simulink model "Clik_Jacobian_inverse_corrado"  (R2023b)
settings: Solver=VariableStepAuto  StartTime=0.0  StopTime=20  RelTol=1e-3
model workspace: external: MAT-File (data not in the file)
undefined symbols (not defined in the file): DiscIntNeverNeededParam, f_s
settings Model: Creator=benit  LastModifiedBy=lalla
settings OptimizationCC: ReuseModelBlockBuffer=off

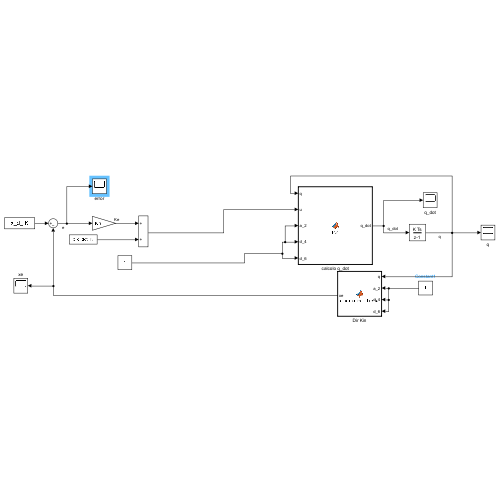
[thumbnail: Simulink's stored preview of the top-level diagram]
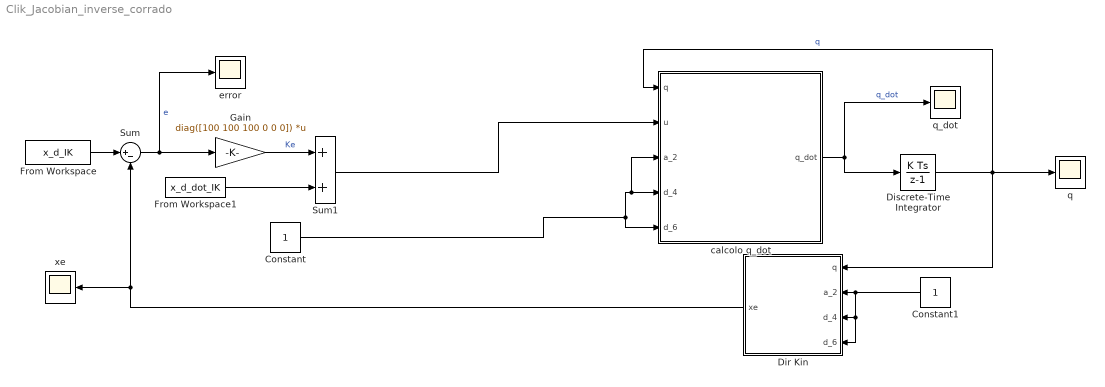
== system Clik_Jacobian_inverse_corrado ==
  Constant : Constant
  Constant1 : Constant
  Dir Kin : MATLAB Function  TreatAsAtomicUnit=on
  Discrete-Time Integrator : DiscreteIntegrator  gainval=1  InitialCondition=[0,0,0,0,0,0]'  SampleTime=1/f_s  ICPrevOutput=DiscIntNeverNeededParam  ICPrevScaledInput=DiscIntNeverNeededParam
  From Workspace : FromWorkspace  VariableName=x_d_IK
  From Workspace1 : FromWorkspace  VariableName=x_d_dot_IK
  Gain : Gain  Gain=diag([100 100 100 0 0 0])  Multiplication=Matrix(K*u)
  Sum : Sum  Inputs=|+-
  Sum1 : Sum
  calcolo q_dot : MATLAB Function  TreatAsAtomicUnit=on
  error : Scope
  q : Scope
  q_dot : Scope
  xe : Scope
  wires:
  Gain/1 -> Sum1/1  "Ke"
  Sum/1 -> error/1, Gain/1  "e"
  From Workspace/1 -> Sum/1
  Discrete-Time Integrator/1 -> q/1, Dir Kin/1(q), calcolo q_dot/1(q)  "q"
  calcolo q_dot/1(q_dot) -> q_dot/1, Discrete-Time Integrator/1  "q_dot"
  Sum1/1 -> calcolo q_dot/2(u)
  Dir Kin/1(xe) -> xe/1, Sum/2
  From Workspace1/1 -> Sum1/2
  Constant/1 -> calcolo q_dot/3(a_2), calcolo q_dot/4(d_4), calcolo q_dot/5(d_6)
  Constant1/1 -> Dir Kin/4(d_6), Dir Kin/3(d_4), Dir Kin/2(a_2)

== matlab function Clik_Jacobian_inverse_corrado/calcolo q_dot ==
  data: q input; u input; a_2 input; d_4 input; q_dot output; d_6 input
function q_dot = fcn(q,u,a_2,d_4,d_6)


theta_1 =q(1);
theta_2 =q(2);
theta_3 =q(3);
theta_4 =q(4);
theta_5 =q(5);
theta_6 =q(6);

    J = [  - d_4*(cos(theta_2)*sin(theta_1)*sin(theta_3) - cos(theta_3)*sin(theta_1)*sin(theta_2)) - d_6*(sin(theta_5)*(cos(theta_1)*sin(theta_4) - cos(theta_4)*(sin(theta_1)*sin(theta_2)*sin(theta_3) - cos(theta_2)*cos(theta_3)*sin(theta_1))) - cos(theta_5)*(cos(theta_2)*sin(theta_1)*sin(theta_3) - cos(theta_3)*sin(theta_1)*sin(theta_2))) - a_2*cos(theta_2)*sin(theta_1),                                                                                           cos(theta_1)*(a_2*sin(theta_2) + d_4*cos(theta_2 - theta_3) + (d_6*sin(theta_2 + theta_3)*sin(theta_4 + theta_5))/2 - (d_6*sin(theta_4 - theta_5)*sin(theta_2 + theta_3))/2 - d_6*cos(theta_2 - theta_3)*cos(theta_5)),                                                                                           cos(theta_1)*(d_4*cos(theta_2 - theta_3) + (d_6*sin(theta_2 + theta_3)*sin(theta_4 + theta_5))/2 - (d_6*sin(theta_4 - theta_5)*sin(theta_2 + theta_3))/2 - d_6*cos(theta_2 - theta_3)*cos(theta_5)), -d_6*sin(theta_5)*(2*cos(theta_3)^2*cos(theta_4)*sin(theta_1) - cos(theta_4)*sin(theta_1) + cos(theta_1)*cos(theta_2)*cos(theta_3)*sin(theta_4) + cos(theta_1)*sin(theta_2)*sin(theta_3)*sin(theta_4)), d_6*cos(theta_1)*cos(theta_2)*sin(theta_3)*sin(theta_5) - d_6*cos(theta_5)*sin(theta_1)*sin(theta_4) + d_6*cos(theta_1)*cos(theta_3)*sin(theta_2)*sin(theta_5) + 2*d_6*cos(theta_3)^2*cos(theta_5)*sin(theta_1)*sin(theta_4) + d_6*cos(theta_1)*cos(theta_4)*cos(theta_5)*sin(theta_2)*sin(theta_3) - 2*d_6*cos(theta_1)*cos(theta_2)*cos(theta_4)^2*sin(theta_3)*sin(theta_5) - 2*d_6*cos(theta_1)*cos(theta_3)*cos(theta_4)^2*sin(theta_2)*sin(theta_5) + d_6*cos(theta_1)*cos(theta_2)*cos(theta_3)*cos(theta_4)*cos(theta_5),                                                                                                                                                                                                                           0;
            d_6*(sin(theta_5)*(sin(theta_1)*sin(theta_4) - cos(theta_4)*(cos(theta_1)*sin(theta_2)*sin(theta_3) - cos(theta_1)*cos(theta_2)*cos(theta_3))) - cos(theta_5)*(cos(theta_1)*cos(theta_2)*sin(theta_3) - cos(theta_1)*cos(theta_3)*sin(theta_2))) + d_4*(cos(theta_1)*cos(theta_2)*sin(theta_3) - cos(theta_1)*cos(theta_3)*sin(theta_2)) + a_2*cos(theta_1)*cos(theta_2),                                                                                          -sin(theta_1)*(a_2*sin(theta_2) + d_4*cos(theta_2 - theta_3) + (d_6*sin(theta_2 + theta_3)*sin(theta_4 + theta_5))/2 - (d_6*sin(theta_4 - theta_5)*sin(theta_2 + theta_3))/2 - d_6*cos(theta_2 - theta_3)*cos(theta_5)),                                                                                          -sin(theta_1)*(d_4*cos(theta_2 - theta_3) + (d_6*sin(theta_2 + theta_3)*sin(theta_4 + theta_5))/2 - (d_6*sin(theta_4 - theta_5)*sin(theta_2 + theta_3))/2 - d_6*cos(theta_2 - theta_3)*cos(theta_5)),  d_6*sin(theta_5)*(2*cos(theta_1)*cos(theta_3)^2*cos(theta_4) - cos(theta_1)*cos(theta_4) + cos(theta_2)*cos(theta_3)*sin(theta_1)*sin(theta_4) + sin(theta_1)*sin(theta_2)*sin(theta_3)*sin(theta_4)), d_6*cos(theta_1)*cos(theta_5)*sin(theta_4) - d_6*cos(theta_2)*sin(theta_1)*sin(theta_3)*sin(theta_5) - d_6*cos(theta_3)*sin(theta_1)*sin(theta_2)*sin(theta_5) - 2*d_6*cos(theta_1)*cos(theta_3)^2*cos(theta_5)*sin(theta_4) - d_6*cos(theta_2)*cos(theta_3)*cos(theta_4)*cos(theta_5)*sin(theta_1) - d_6*cos(theta_4)*cos(theta_5)*sin(theta_1)*sin(theta_2)*sin(theta_3) + 2*d_6*cos(theta_2)*cos(theta_4)^2*sin(theta_1)*sin(theta_3)*sin(theta_5) + 2*d_6*cos(theta_3)*cos(theta_4)^2*sin(theta_1)*sin(theta_2)*sin(theta_5),                                                                                                                                                                                                                             0;
                                                                                                                                                                                                                                                                                                                                                                        0, -cos(2*theta_1)*(a_2*cos(theta_2) + d_4*cos(theta_2)*sin(theta_3) - d_4*cos(theta_3)*sin(theta_2) - d_6*cos(theta_2)*cos(theta_5)*sin(theta_3) + d_6*cos(theta_3)*cos(theta_5)*sin(theta_2) + d_6*cos(theta_2)*cos(theta_3)*cos(theta_4)*sin(theta_5) - d_6*cos(theta_4)*sin(theta_2)*sin(theta_3)*sin(theta_5)), -cos(2*theta_1)*(d_4*cos(theta_2)*sin(theta_3) - d_4*cos(theta_3)*sin(theta_2) - d_6*cos(theta_2)*cos(theta_5)*sin(theta_3) + d_6*cos(theta_3)*cos(theta_5)*sin(theta_2) + d_6*cos(theta_2)*cos(theta_3)*cos(theta_4)*sin(theta_5) - d_6*cos(theta_4)*sin(theta_2)*sin(theta_3)*sin(theta_5)),                                                                                                                                   -d_6*sin(theta_2 - theta_3)*cos(2*theta_1)*sin(theta_4)*sin(theta_5),                                                                                                                                                                                             d_6*cos(2*theta_1)*(sin(theta_2)*sin(theta_3)*sin(theta_5) - cos(theta_2)*cos(theta_3)*sin(theta_5) + 2*cos(theta_2)*cos(theta_3)*cos(theta_4)^2*sin(theta_5) - 2*cos(theta_4)^2*sin(theta_2)*sin(theta_3)*sin(theta_5) - cos(theta_2)*cos(theta_4)*cos(theta_5)*sin(theta_3) + cos(theta_3)*cos(theta_4)*cos(theta_5)*sin(theta_2)),                                                                                                                                                                                                                                          0;
                                                                                                                                                                                                                                                                                                                                                              0,                                                                                                                                                                                                                                                                                                     sin(theta_1),                                                                                                                                                                                                                                                                                  sin(theta_1),                                                                                                                                                                   -sin(theta_2 - theta_3)*cos(theta_1),                                                                                                                                                                                                                                                                                                                                                                                                       sin(theta_4)*(cos(theta_1)*sin(theta_2)*sin(theta_3) - cos(theta_1)*cos(theta_2)*cos(theta_3)) - cos(theta_4)*sin(theta_1), sin(theta_5)*(sin(theta_1)*sin(theta_4) - cos(theta_4)*(cos(theta_1)*sin(theta_2)*sin(theta_3) - cos(theta_1)*cos(theta_2)*cos(theta_3))) - cos(theta_5)*(cos(theta_1)*cos(theta_2)*sin(theta_3) - cos(theta_1)*cos(theta_3)*sin(theta_2));
                                                                                                                                                                                                                                                                                                                                                                         0,                                                                                                                                                                                                                                                                                                     cos(theta_1),                                                                                                                                                                                                                                                                                  cos(theta_1),                                                                                                                                                                   -sin(theta_2 - theta_3)*sin(theta_1),                                                                                                                                                                                                                                                                                                                                                                                                       sin(theta_4)*(sin(theta_1)*sin(theta_2)*sin(theta_3) - cos(theta_2)*cos(theta_3)*sin(theta_1)) - cos(theta_1)*cos(theta_4), sin(theta_5)*(cos(theta_1)*sin(theta_4) - cos(theta_4)*(sin(theta_1)*sin(theta_2)*sin(theta_3) - cos(theta_2)*cos(theta_3)*sin(theta_1))) - cos(theta_5)*(cos(theta_2)*sin(theta_1)*sin(theta_3) - cos(theta_3)*sin(theta_1)*sin(theta_2));
                                                                                                                                                                                                                                                                                                                                                              1,                                                                                                                                                                                                                                                                                                                0,                                                                                                                                                                                                                                                                                             0,                                                                                                                                                                                 cos(theta_2 - theta_3),                                                                                                                                                                                                                                                                                                                                                                                                                                                                                             -sin(theta_2 + theta_3)*sin(theta_4),                                                                                                                                                     sin(theta_2 + theta_3)*cos(theta_4)*sin(theta_5) - cos(theta_2 - theta_3)*cos(theta_5)];
 
    q_dot = pinv(J)*u;

end

== matlab function Clik_Jacobian_inverse_corrado/Dir Kin ==
  data: q input; xe output; a_2 input; d_4 input; d_6 input
function xe = cinematica_diretta(q,a_2,d_4,d_6)
 
theta_1 =q(1);
theta_2 =q(2);
theta_3 =q(3);
theta_4 =q(4);
theta_5 =q(5);
theta_6 =q(6);


Te=[cos(theta_6)*(cos(theta_5)*(sin(theta_1)*sin(theta_4) - cos(theta_4)*(cos(theta_1)*sin(theta_2)*sin(theta_3) - cos(theta_1)*cos(theta_2)*cos(theta_3))) - sin(theta_5)*(cos(theta_1)*cos(theta_2)*sin(theta_3) - cos(theta_1)*cos(theta_3)*sin(theta_2))) - sin(theta_6)*(cos(theta_4)*sin(theta_1) - sin(theta_4)*(cos(theta_1)*sin(theta_2)*sin(theta_3) - cos(theta_1)*cos(theta_2)*cos(theta_3))), - cos(theta_6)*(cos(theta_4)*sin(theta_1) - sin(theta_4)*(cos(theta_1)*sin(theta_2)*sin(theta_3) - cos(theta_1)*cos(theta_2)*cos(theta_3))) - sin(theta_6)*(cos(theta_5)*(sin(theta_1)*sin(theta_4) - cos(theta_4)*(cos(theta_1)*sin(theta_2)*sin(theta_3) - cos(theta_1)*cos(theta_2)*cos(theta_3))) - sin(theta_5)*(cos(theta_1)*cos(theta_2)*sin(theta_3) - cos(theta_1)*cos(theta_3)*sin(theta_2))), sin(theta_5)*(sin(theta_1)*sin(theta_4) - cos(theta_4)*(cos(theta_1)*sin(theta_2)*sin(theta_3) - cos(theta_1)*cos(theta_2)*cos(theta_3))) - cos(theta_5)*(cos(theta_1)*cos(theta_2)*sin(theta_3) - cos(theta_1)*cos(theta_3)*sin(theta_2)), d_6*(sin(theta_5)*(sin(theta_1)*sin(theta_4) - cos(theta_4)*(cos(theta_1)*sin(theta_2)*sin(theta_3) - cos(theta_1)*cos(theta_2)*cos(theta_3))) - cos(theta_5)*(cos(theta_1)*cos(theta_2)*sin(theta_3) - cos(theta_1)*cos(theta_3)*sin(theta_2))) + d_4*(cos(theta_1)*cos(theta_2)*sin(theta_3) - cos(theta_1)*cos(theta_3)*sin(theta_2)) + a_2*cos(theta_1)*cos(theta_2);
    cos(theta_6)*(cos(theta_5)*(cos(theta_1)*sin(theta_4) - cos(theta_4)*(sin(theta_1)*sin(theta_2)*sin(theta_3) - cos(theta_2)*cos(theta_3)*sin(theta_1))) - sin(theta_5)*(cos(theta_2)*sin(theta_1)*sin(theta_3) - cos(theta_3)*sin(theta_1)*sin(theta_2))) - sin(theta_6)*(cos(theta_1)*cos(theta_4) - sin(theta_4)*(sin(theta_1)*sin(theta_2)*sin(theta_3) - cos(theta_2)*cos(theta_3)*sin(theta_1))), - cos(theta_6)*(cos(theta_1)*cos(theta_4) - sin(theta_4)*(sin(theta_1)*sin(theta_2)*sin(theta_3) - cos(theta_2)*cos(theta_3)*sin(theta_1))) - sin(theta_6)*(cos(theta_5)*(cos(theta_1)*sin(theta_4) - cos(theta_4)*(sin(theta_1)*sin(theta_2)*sin(theta_3) - cos(theta_2)*cos(theta_3)*sin(theta_1))) - sin(theta_5)*(cos(theta_2)*sin(theta_1)*sin(theta_3) - cos(theta_3)*sin(theta_1)*sin(theta_2))), sin(theta_5)*(cos(theta_1)*sin(theta_4) - cos(theta_4)*(sin(theta_1)*sin(theta_2)*sin(theta_3) - cos(theta_2)*cos(theta_3)*sin(theta_1))) - cos(theta_5)*(cos(theta_2)*sin(theta_1)*sin(theta_3) - cos(theta_3)*sin(theta_1)*sin(theta_2)), d_4*(cos(theta_2)*sin(theta_1)*sin(theta_3) - cos(theta_3)*sin(theta_1)*sin(theta_2)) + d_6*(sin(theta_5)*(cos(theta_1)*sin(theta_4) - cos(theta_4)*(sin(theta_1)*sin(theta_2)*sin(theta_3) - cos(theta_2)*cos(theta_3)*sin(theta_1))) - cos(theta_5)*(cos(theta_2)*sin(theta_1)*sin(theta_3) - cos(theta_3)*sin(theta_1)*sin(theta_2))) + a_2*cos(theta_2)*sin(theta_1);
                                                                                                                                                                                                                                          - cos(theta_6)*(cos(theta_2 - theta_3)*sin(theta_5) - sin(theta_2 + theta_3)*cos(theta_4)*cos(theta_5)) - sin(theta_2 + theta_3)*sin(theta_4)*sin(theta_6),                                                                                                                                                                                                                                                sin(theta_6)*(cos(theta_2 - theta_3)*sin(theta_5) - sin(theta_2 + theta_3)*cos(theta_4)*cos(theta_5)) - sin(theta_2 + theta_3)*cos(theta_6)*sin(theta_4),                                                                                                                                                     sin(theta_2 + theta_3)*cos(theta_4)*sin(theta_5) - cos(theta_2 - theta_3)*cos(theta_5),                                                                                                                                                                  a_2*sin(theta_2) + d_4*cos(theta_2 - theta_3) + (d_6*sin(theta_2 + theta_3)*sin(theta_4 + theta_5))/2 - (d_6*sin(theta_4 - theta_5)*sin(theta_2 + theta_3))/2 - d_6*cos(theta_2 - theta_3)*cos(theta_5);
                                                                                                                                                                                                                                                                                                                                                                                                    0,                                                                                                                                                                                                                                                                                                                                                                                                       0,                                                                                                                                                                                                                                          0,                                                                                                                                                                                                                                                                                                                                                                        1];
phy=atan2(Te(2,1),Te(1,1));
theta=atan2(-Te(3,1),sqrt(Te(3,2)^2+Te(3,3)^2));
psy=atan2(Te(3,2),Te(3,3));

xe= [Te(1:3,4);phy;theta;psy];
 
end
